simulink model "test_env"  (R2019b)
settings: Solver=FixedStepAuto  StartTime=0.0  StopTime=30  FixedStep=0.01  RelTol=1e-3
values from neighbouring files (symbols this model uses):
  dT = dT2    [SCARSSetup.m]    (also in plot_position.m = 1; pwsat2_setup.m = 5; scars_setup.m = 0.01; startup.m = 1)
  initDay = 0    [SCARSSetup.m]    (also in pwsat2_setup.m; pwsat2_tle.m; scars_setup.m)
  initYear = 2000    [SCARSSetup.m]    (also in pwsat2_setup.m; pwsat2_tle.m; scars_setup.m)
  Re = 6356e3    (= 6356000)    [SCARSSetup.m]    (also in pwsat2_setup.m; pwsat2_tle.m; scars_setup.m; startup.m)
  sun_position = getSunPositions(julian, TFinal, dT)    [SCARSSetup.m]    (also in pwsat2_setup.m; scars_setup.m)
  TFinal = 5    [plot_eci2ecef.m]    (also in plot_position.m = 1500; pwsat2_setup.m = 1728000; scars_setup.m = 100)
undefined symbols (not defined in the file or in its folder): m_bias, st_ex_earth, st_ex_sun, st_lost, st_vector
libraries: scars_library x9, simulink_extras x8, aerolibutil x3, aerolibatmos2 x2, sharedtransform x2, vrlib x1, simulink x1
settings Model: Creator=asmialek  LastModifiedBy=asmialek

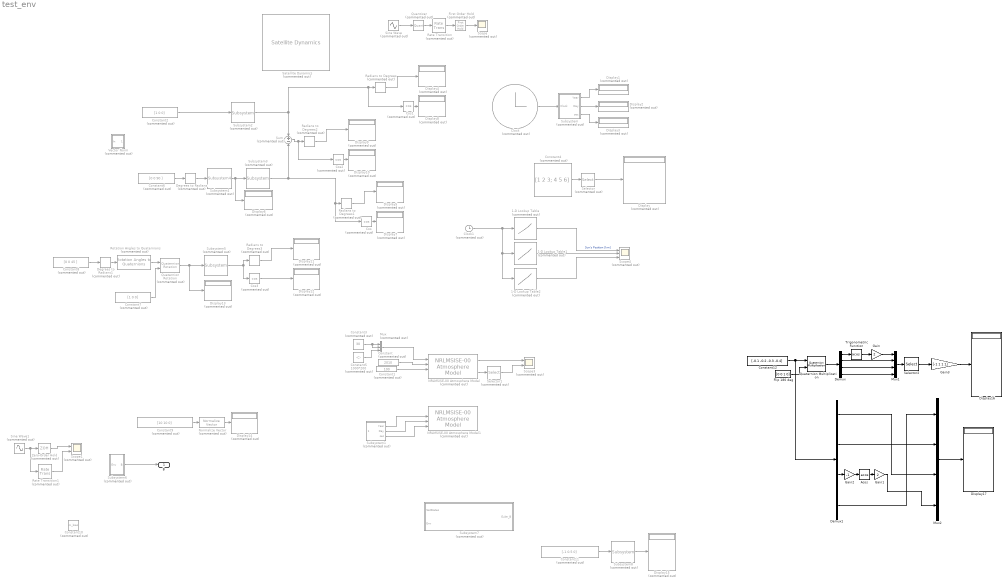
== system test_env ==
  1-D Lookup Table : Lookup_n-D  Commented=on  NumberOfTableDimensions=1  BreakpointsForDimension1=[0:dT:TFinal]  Table=sun_position(:,1)  InternalRulePriority=Speed  RndMeth=Simplest  InputSameDT=on
  1-D Lookup Table1 : Lookup_n-D  Commented=on  NumberOfTableDimensions=1  BreakpointsForDimension1=[0:dT:TFinal]  Table=sun_position(:,2)  InternalRulePriority=Speed  RndMeth=Simplest  InputSameDT=on
  1-D Lookup Table2 : Lookup_n-D  Commented=on  NumberOfTableDimensions=1  BreakpointsForDimension1=[0:dT:TFinal]  Table=sun_position(:,3)  InternalRulePriority=Speed  RndMeth=Simplest  InputSameDT=on
  Acos : Trigonometry  Operator=acos
  Clock : Clock  Commented=on
      settings: Decimation=100
  Clock1 : Clock  Commented=on
  Constant : Constant  Commented=on  Value=2010
  Constant1 : Constant  Commented=on  Value=100
  Constant10 : Constant  Commented=on  Value=m_bias
  Constant11 : Constant  Commented=on  Value=[-1 0.5 0]
  Constant12 : Constant  Value=[-0.1 -0.2 -0.3 -0.4]
  Constant2 : Constant  Commented=on  Value=[1 0 0]
  Constant3 : Constant  Commented=on  Value=30
  Constant4 : Constant  Commented=on  Value=[1 2 3; 4 5 6]
  Constant5 : Constant  Commented=on  Value=1000*200
  Constant6 : Constant  Commented=on  Value=[0 0 90 ]
  Constant7 : Constant  Commented=on  Value=[1 0 0]
  Constant8 : Constant  Commented=on  Value=[0 0 45 ]
  Constant9 : Constant  Commented=on  Value=[10 10 0]
  Cos{,1..3} (4 alike) : Trigonometry  Commented=on  Operator=cos
  Degrees to Radians : simulink_extras/Transformations/Degrees to Radians  Commented=on
  Degrees to Radians1 : simulink_extras/Transformations/Degrees to Radians  Commented=on
  Demux : Demux
  Demux1 : Demux
  Display{,1..15} (16 alike) : Display  Commented=on
  Display16 : Display
  Display17 : Display
  First Order Hold : FirstOrderHold  Commented=on  ErrorTolerance=inf
  Flip 180 deg : Constant  Value=[0 0 1 0]
  Gain : Gain  Gain=2
  Gain1 : Gain  Gain=2
  Gain2 : Gain  Gain=-1
  Gain3 : Gain  Gain=[-1 1 1 1]
  Mux : Mux  Commented=on  Inputs=3
  Mux1 : Mux
  Mux2 : Mux
  NRLMSISE-00 Atmosphere Model : aerolibatmos2/NRLMSISE-00 Atmosphere Model  Commented=on  units=Metric (MKS)  lst_input=off  flux_ap_input=off  flags_input=Internal  flags=ones(1,23)  oxygen_in=off  action=Warning
      settings: SourceProductName=Aerospace Blockset  SourceProductBaseCode=AE
  NRLMSISE-00 Atmosphere Model1 : aerolibatmos2/NRLMSISE-00 Atmosphere Model  Commented=on  units=Metric (MKS)  lst_input=off  flux_ap_input=off  flags_input=Internal  flags=ones(1,23)  oxygen_in=off  action=Warning
      settings: SourceProductName=Aerospace Blockset  SourceProductBaseCode=AE
  Normalize Vector : vrlib/Utilities/Normalize Vector  Commented=on  maxzero=0
      settings: SourceProductName=Simulink
  Quantizer : Quantizer  Commented=on  QuantizationInterval=0.01
  Quaternion Multiplication : aerolibutil/Quaternion Multiplication
  Quaternion Rotation : aerolibutil/Quaternion Rotation  Commented=on
  Radians to Degrees{,1..3} (4 alike) : simulink_extras/Transformations/Radians to Degrees  Commented=on
  Rate Transition : RateTransition  Commented=on  OutPortSampleTime=0.1
  Rate Transition1 : RateTransition  Commented=on  OutPortSampleTime=0.3
  Rotation Angles to Quaternions : sharedtransform/Rotation Angles to Quaternions  Commented=on  rotationOrder=XYZ  aMode=aMode
      settings: SourceProductName=Aerospace Blockset  SourceProductBaseCode=AE
  Satellite Dynamics : scars_library/Advanced/Satellite Dynamics  Commented=on  Parameter4=Keplerian Elements  epoch=0  mass=0  a=6356e3+400e3  e=0  incl=0  RA=0  w=0  TA=0  initEuler=[0 0 0]  initEulerRates=[0 0 0]  TA_copy=0  TA_copy_copy=0  TA_copy_copy_copy=[10 25]  TA_copy_copy_copy_copy=[10 25]  initEuler_copy=[0 0 0]  initEulerRates_copy=[0 0 0]
  Scope : Scope  Commented=on
  Scope1 : Scope  Commented=on  NumInputPorts=2
  Scope3 : Scope  Commented=on  NumInputPorts=2
  Scope4 : Scope  Commented=on  NumInputPorts=3
  Selector : Selector  Commented=on  NumberOfDimensions=2  InputPortWidth=2  IndexOptions=Index vector (dialog),Select all  Indices=1,3  OutputSizes=1,1
  Selector1 : Selector  Commented=on  InputPortWidth=9  IndexOptions=Index vector (dialog)  Indices=6  OutputSizes=1
  Selector2 : Selector  InputPortWidth=4  IndexOptions=Index vector (dialog)  Indices=[2 4 3 1]  OutputSizes=1
  Sine Wave : Sin  Commented=on  SampleTime=0
  Sine Wave1 : Sin  Commented=on  SampleTime=0
  Subsystem : Subsystem  Commented=on
  Subsystem1 : Subsystem  Commented=on
  Subsystem{2..3,5,8} (4 alike) : scars_library/Subsystem  Commented=on  SystemSampleTime=-1  Latency=0  AutoFrameSizeCalculation=off
  Subsystem4 : scars_library/Subsystem4  Commented=on  SystemSampleTime=-1  Latency=0  AutoFrameSizeCalculation=off
  Subsystem6 : Subsystem  Commented=on  mask{m_power=0.1, m_freq=10, m_bias=[0.01 0.01 0.01]}
      mask prompts: m_power "Noise Power Spectral Density"; m_freq "Sampling Frequncy [Hz]"; m_bias "Measurement Bias [nT]"
  Subsystem7 : Subsystem  Commented=on
  Sum : Sum  Commented=on  Inputs=+|-
  Trigonometric Function : Trigonometry  Operator=acos
  Vector Norm : Subsystem  Commented=on
  Zero-Order Hold : ZeroOrderHold  Commented=on  SampleTime=0.3
  B : Outport
  wires:
  Sine Wave/1 -> Quantizer/1
  Quantizer/1 -> Rate Transition/1
  First Order Hold/1 -> Scope/1
  Rate Transition/1 -> First Order Hold/1
  Constant/1 -> NRLMSISE-00 Atmosphere Model/2
  Constant1/1 -> NRLMSISE-00 Atmosphere Model/3
  NRLMSISE-00 Atmosphere Model/1 -> Scope3/1
  Mux/1 -> NRLMSISE-00 Atmosphere Model/1
  Constant3/1 -> Mux/1, Mux/2
  Clock1/1 -> 1-D Lookup Table2/1, 1-D Lookup Table1/1, 1-D Lookup Table/1
  1-D Lookup Table/1 -> Scope4/1  "Sun's Position [km]"
  1-D Lookup Table1/1 -> Scope4/2
  1-D Lookup Table2/1 -> Scope4/3
  Selector/1 -> Display/1
  Constant4/1 -> Selector/1
  NRLMSISE-00 Atmosphere Model/2 -> Selector1/1
  Selector1/1 -> Scope3/2
  Constant5/1 -> Mux/3
  Subsystem/1(Year) -> Display1/1
  Subsystem/3(sec) -> Display3/1
  Subsystem/2(Day) -> Display2/1
  Clock/1 -> Subsystem/1(Clock)
  Subsystem1/1(Year) -> NRLMSISE-00 Atmosphere Model1/2
  Subsystem1/2(Day) -> NRLMSISE-00 Atmosphere Model1/3
  Subsystem1/3(sec) -> NRLMSISE-00 Atmosphere Model1/4
  Constant2/1 -> Subsystem2/1
  Subsystem2/1 -> Sum/1, Cos1/1, Radians to Degrees/1
  Constant6/1 -> Degrees to Radians/1
  Subsystem3/1 -> Cos/1, Radians to Degrees1/1, Sum/2
  Radians to Degrees1/1 -> Display5/1
  Subsystem4/1 -> Subsystem3/1, Display6/1
  Cos/1 -> Display7/1
  Cos1/1 -> Display8/1
  Radians to Degrees/1 -> Display4/1
  Degrees to Radians/1 -> Subsystem4/1
  Cos2/1 -> Display10/1
  Radians to Degrees2/1 -> Display9/1
  Sum/1 -> Cos2/1, Radians to Degrees2/1
  Rotation Angles to Quaternions/1 -> Quaternion Rotation/1
  Constant8/1 -> Degrees to Radians1/1
  Degrees to Radians1/1 -> Rotation Angles to Quaternions/1
  Constant7/1 -> Quaternion Rotation/2
  Radians to Degrees3/1 -> Display11/1
  Subsystem5/1 -> Radians to Degrees3/1, Cos3/1
  Cos3/1 -> Display12/1
  Quaternion Rotation/1 -> Display13/1, Subsystem5/1
  Constant9/1 -> Normalize Vector/1
  Normalize Vector/1 -> Display14/1
  Sine Wave1/1 -> Rate Transition1/1, Zero-Order Hold/1
  Rate Transition1/1 -> Scope1/2
  Zero-Order Hold/1 -> Scope1/1
  Subsystem6/1(B) -> B/1
  ? -> Subsystem6/1(Env)
  Subsystem8/1 -> Display15/1
  Constant11/1 -> Subsystem8/1
  Quaternion Multiplication/1 -> Demux/1
  Selector2/1 -> Gain3/1
  Mux1/1 -> Selector2/1
  Gain/1 -> Mux1/1
  Demux/1 -> Trigonometric Function/1
  Demux/3 -> Mux1/3
  Demux/2 -> Mux1/2
  Trigonometric Function/1 -> Gain/1
  Flip 180 deg/1 -> Quaternion Multiplication/2
  Demux/4 -> Mux1/4
  Gain3/1 -> Display16/1
  Demux1/4 -> Mux2/1
  Gain2/1 -> Acos/1
  Gain1/1 -> Mux2/4
  Acos/1 -> Gain1/1
  Demux1/3 -> Gain2/1
  Demux1/2 -> Mux2/2
  Constant12/1 -> Demux1/1, Quaternion Multiplication/1
  Demux1/1 -> Mux2/3
  Mux2/1 -> Display17/1

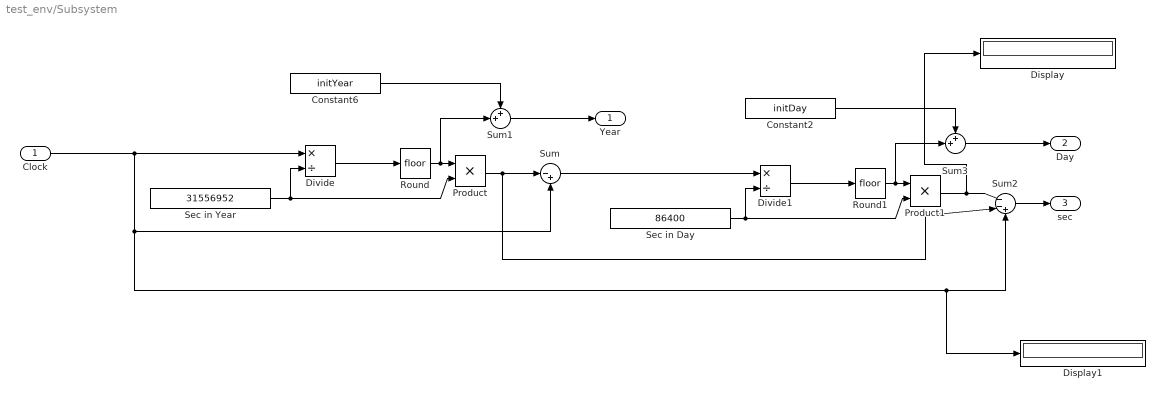
== system test_env/Subsystem ==
  Clock : Inport
  Constant2 : Constant  Value=initDay
  Constant6 : Constant  Value=initYear
  Display : Display
  Display1 : Display
  Divide : Product  Inputs=*/
  Divide1 : Product  Inputs=*/
  Product : Product
  Product1 : Product
  Round : Rounding
  Round1 : Rounding
  Sec in Day : Constant  Value=86400
  Sec in Year : Constant  Value=31556952
  Sum : Sum  Inputs=|-+
  Sum1 : Sum  Inputs=++|
  Sum2 : Sum  Inputs=|--+
  Sum3 : Sum  Inputs=++|
  Year : Outport
  Day : Outport  Port=2
  sec : Outport  Port=3
  wires:
  Sum1/1 -> Year/1
  Sum3/1 -> Day/1
  Round1/1 -> Sum3/2, Product1/1
  Sum2/1 -> sec/1
  Product/1 -> Sum2/2, Sum/1
  Round/1 -> Sum1/2, Product/1
  Sum/1 -> Divide1/1
  Divide1/1 -> Round1/1
  Product1/1 -> Display/1, Sum2/1
  Sec in Day/1 -> Product1/2, Divide1/2
  Constant2/1 -> Sum3/1
  Sec in Year/1 -> Product/2, Divide/2
  Divide/1 -> Round/1
  Clock/1 -> Divide/1, Display1/1, Sum2/3, Sum/2
  Constant6/1 -> Sum1/1

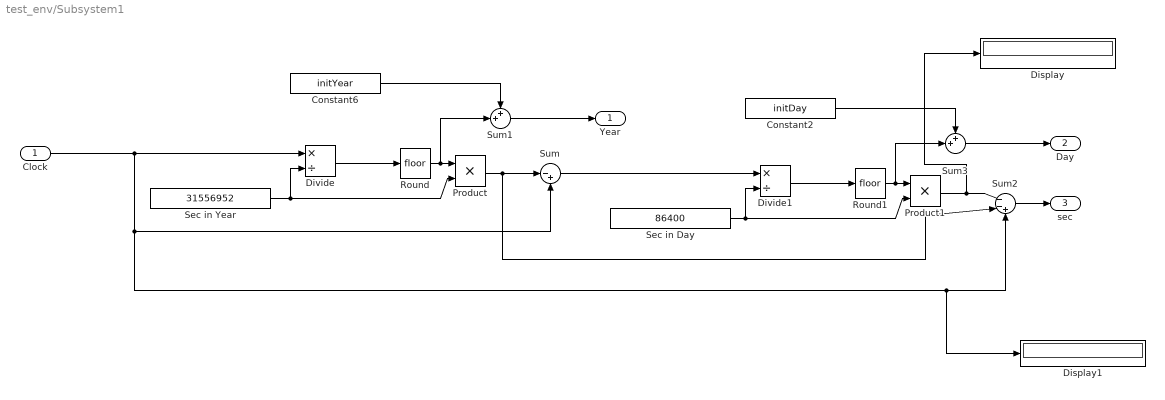
== system test_env/Subsystem1 ==
  Clock : Inport
  Constant2 : Constant  Value=initDay
  Constant6 : Constant  Value=initYear
  Display : Display
  Display1 : Display
  Divide : Product  Inputs=*/
  Divide1 : Product  Inputs=*/
  Product : Product
  Product1 : Product
  Round : Rounding
  Round1 : Rounding
  Sec in Day : Constant  Value=86400
  Sec in Year : Constant  Value=31556952
  Sum : Sum  Inputs=|-+
  Sum1 : Sum  Inputs=++|
  Sum2 : Sum  Inputs=|--+
  Sum3 : Sum  Inputs=++|
  Year : Outport
  Day : Outport  Port=2
  sec : Outport  Port=3
  wires:
  Sum1/1 -> Year/1
  Sum3/1 -> Day/1
  Round1/1 -> Sum3/2, Product1/1
  Sum2/1 -> sec/1
  Product/1 -> Sum2/2, Sum/1
  Round/1 -> Sum1/2, Product/1
  Sum/1 -> Divide1/1
  Divide1/1 -> Round1/1
  Product1/1 -> Display/1, Sum2/1
  Sec in Day/1 -> Product1/2, Divide1/2
  Constant2/1 -> Sum3/1
  Sec in Year/1 -> Product/2, Divide/2
  Divide/1 -> Round/1
  Clock/1 -> Divide/1, Display1/1, Sum2/3, Sum/2
  Constant6/1 -> Sum1/1

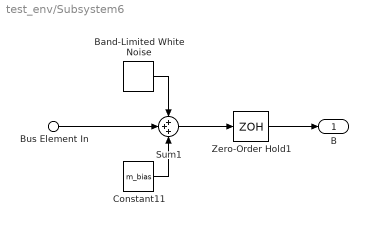
== system test_env/Subsystem6 ==
  Bus Element In : Inport  PortName=Env  Element=Magnetic Field [nT]
  Band-Limited White Noise : simulink/Sources/Band-Limited White Noise  Cov=m_power*[1 1 1]  Ts=1/m_freq  seed="[ randi(1000, 1, 3)  ]"
  Constant11 : Constant  Value=m_bias
  Sum1 : Sum  Inputs=+++
  Zero-Order Hold1 : ZeroOrderHold  SampleTime=1/m_freq
  B : Outport
  wires:
  Constant11/1 -> Sum1/3
  Bus Element In/1 -> Sum1/2
  Zero-Order Hold1/1 -> B/1
  Band-Limited White Noise/1 -> Sum1/1
  Sum1/1 -> Zero-Order Hold1/1

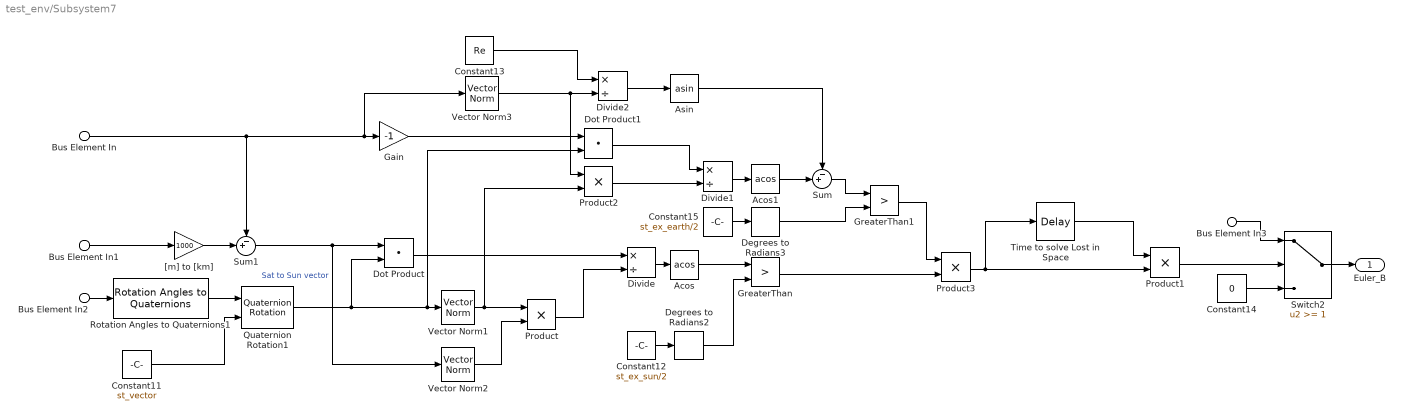
== system test_env/Subsystem7 ==
  Bus Element In : Inport  PortName=SatStates  Element=X_ecef
  Bus Element In2 : Inport  PortName=SatStates  Element=Euler_B
  Bus Element In3 : Inport  PortName=SatStates  Element=Euler_B
  Bus Element In1 : Inport  Port=2  PortName=Env  Element=Sun's Position [km]
  Acos : Trigonometry  Operator=acos
  Acos1 : Trigonometry  Operator=acos
  Asin : Trigonometry  Operator=asin
  Constant11 : Constant  Value=st_vector
  Constant12 : Constant  Value=st_ex_sun/2
  Constant13 : Constant  Value=Re
  Constant14 : Constant  Value=0
  Constant15 : Constant  Value=st_ex_earth/2
  Degrees to Radians2 : simulink_extras/Transformations/Degrees to Radians
  Degrees to Radians3 : simulink_extras/Transformations/Degrees to Radians
  Divide : Product  Inputs=*/
  Divide1 : Product  Inputs=*/
  Divide2 : Product  Inputs=*/
  Dot Product : DotProduct  InputSameDT=on  OutDataTypeStr=Inherit: Inherit via internal rule
  Dot Product1 : DotProduct  InputSameDT=on  OutDataTypeStr=Inherit: Inherit via internal rule
  Gain : Gain  Gain=-1
  GreaterThan : RelationalOperator  Operator=>  OutDataTypeStr=boolean  RndMeth=Simplest
  GreaterThan1 : RelationalOperator  Operator=>  OutDataTypeStr=boolean  RndMeth=Simplest
  Product{,1..3} (4 alike) : Product
  Quaternion Rotation1 : aerolibutil/Quaternion Rotation
  Rotation Angles to Quaternions1 : sharedtransform/Rotation Angles to Quaternions  rotationOrder=XYZ  aMode=aMode
      settings: SourceProductName=Aerospace Blockset  SourceProductBaseCode=AE
  Sum : Sum  Inputs=-+|
  Sum1 : Sum  Inputs=-+|
  Switch2 : Switch  Threshold=1
  Time to solve Lost in Space : TransportDelay  DelayTime=st_lost  InitialOutput=1
  Vector Norm1 : scars_library/Vector Norm  SystemSampleTime=-1  Latency=0  AutoFrameSizeCalculation=off
  Vector Norm2 : scars_library/Vector Norm  SystemSampleTime=-1  Latency=0  AutoFrameSizeCalculation=off
  Vector Norm3 : scars_library/Vector Norm  SystemSampleTime=-1  Latency=0  AutoFrameSizeCalculation=off
  "[m] to [km]" : Gain  Gain=1000
  Euler_B : Outport
  wires:
  GreaterThan1/1 -> Product3/1
  Rotation Angles to Quaternions1/1 -> Quaternion Rotation1/1
  Bus Element In/1 -> Sum1/1, Vector Norm3/1, Gain/1
  Acos/1 -> GreaterThan/1
  Constant13/1 -> Divide2/1
  "[m] to [km]"/1 -> Sum1/2
  Quaternion Rotation1/1 -> Dot Product/2, Dot Product1/2, Vector Norm1/1
  Vector Norm1/1 -> Product2/2, Product/1
  Product/1 -> Divide/2
  Switch2/1 -> Euler_B/1
  Bus Element In2/1 -> Rotation Angles to Quaternions1/1
  Product1/1 -> Switch2/2
  Product3/1 -> Product1/2, Time to solve Lost in Space/1
  Constant15/1 -> Degrees to Radians3/1
  Degrees to Radians3/1 -> GreaterThan1/2
  GreaterThan/1 -> Product3/2
  Constant14/1 -> Switch2/3
  Vector Norm3/1 -> Product2/1, Divide2/2
  Time to solve Lost in Space/1 -> Product1/1
  Sum1/1 -> Vector Norm2/1, Dot Product/1  "Sat to Sun vector"
  Degrees to Radians2/1 -> GreaterThan/2
  Product2/1 -> Divide1/2
  Dot Product/1 -> Divide/1
  Constant11/1 -> Quaternion Rotation1/2
  Divide2/1 -> Asin/1
  Bus Element In3/1 -> Switch2/1
  Constant12/1 -> Degrees to Radians2/1
  Dot Product1/1 -> Divide1/1
  Gain/1 -> Dot Product1/1
  Divide1/1 -> Acos1/1
  Divide/1 -> Acos/1
  Bus Element In1/1 -> "[m] to [km]"/1
  Vector Norm2/1 -> Product/2
  Acos1/1 -> Sum/2
  Sum/1 -> GreaterThan1/1
  Asin/1 -> Sum/1

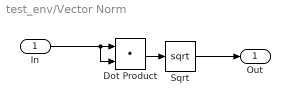
== system test_env/Vector Norm ==
  In : Inport
  Dot Product : DotProduct  InputSameDT=on  OutDataTypeStr=Inherit: Inherit via internal rule
  Sqrt : Sqrt  SaturateOnIntegerOverflow=on
  Out : Outport
  wires:
  In/1 -> Dot Product/2, Dot Product/1
  Dot Product/1 -> Sqrt/1
  Sqrt/1 -> Out/1
